simulink model "manning_test_nonlinear"  (R2022b)
settings: Solver=VariableStepAuto  StartTime=0.0  StopTime=5*N  RelTol=1e-3
undefined symbols (not defined in the file or in its folder): yd_ds
settings Model: Creator=chuan  LastModifiedBy=chuan

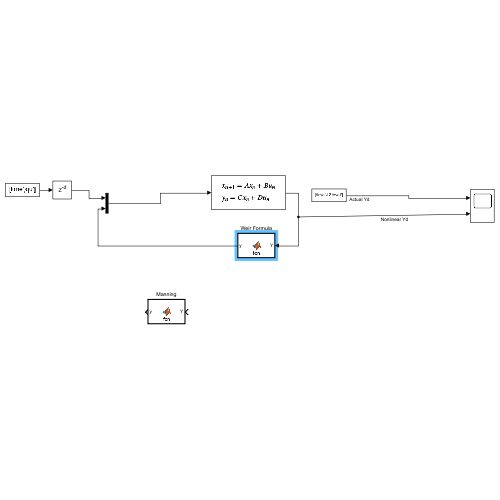
[thumbnail: Simulink's stored preview of the top-level diagram]
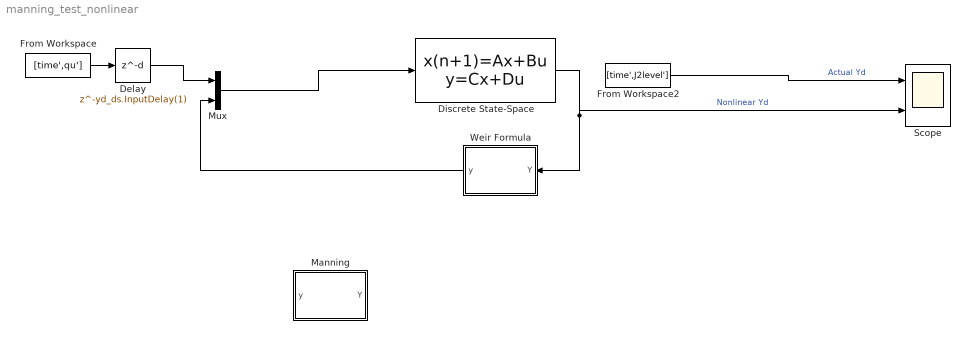
== system manning_test_nonlinear ==
  Delay : Delay  DelayLength=yd_ds.InputDelay(1)  InitialCondition=0
  Discrete State-Space : DiscreteStateSpace  A=yd_ds.A  B=yd_ds.B  C=yd_ds.C  D=yd_ds.D  SampleTime=yd_ds.Ts
  From Workspace : FromWorkspace  VariableName=[time',qu']
  From Workspace2 : FromWorkspace  VariableName=[time',J2level']
  Manning : MATLAB Function  TreatAsAtomicUnit=on
  Mux : Mux  Inputs=2
  Scope : Scope  NumInputPorts=2
  Weir Formula : MATLAB Function  TreatAsAtomicUnit=on
  wires:
  Discrete State-Space/1 -> Scope/2, Weir Formula/1(Y)  "Nonlinear Yd"
  Weir Formula/1(y) -> Mux/2
  Mux/1 -> Discrete State-Space/1
  From Workspace2/1 -> Scope/1  "Actual Yd"
  From Workspace/1 -> Delay/1
  Delay/1 -> Mux/1

== matlab function manning_test_nonlinear/Manning ==
  data: Y input; y output
function y = fcn(Y)
n = 0.02;
Sb = 0.0008;
B=8;
m = 1.5;

Y = max(Y,0);

y = (1/n)*(B*Y + m*Y.^2)*((B*Y + m*Y.^2)/(B + 2.*Y.*sqrt(1+m^2))).^(2/3) .* sqrt(Sb);

== matlab function manning_test_nonlinear/Weir Formula ==
  data: Y input; y output
function y = fcn(Y)
% Downstream_Area = 2720;
Yfull = 40;
A0 = 2720;
Cd = 1;
g = 9.81;

Y = max(Y,0);

CwL = (Cd*A0*sqrt(g))/(Yfull);
y = CwL*((Y)^(1.5));
